simulink model "DriveFinal"  (R2023a)
settings: Solver=FixedStepDiscrete  StartTime=0.0  StopTime=10.0  FixedStep=0.01  RelTol=1e-3
undefined symbols (not defined in the file): InputPWM, WheelSpeed
libraries: mobileRoboticsTrainingLib x5
settings Model: Creator=Jack Youens  LastModifiedBy=jakew

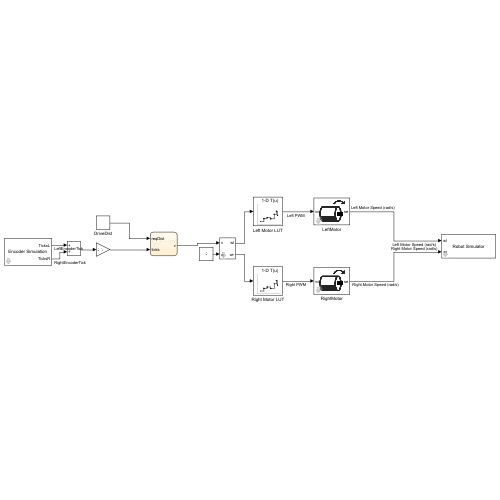
[thumbnail: Simulink's stored preview of the top-level diagram]
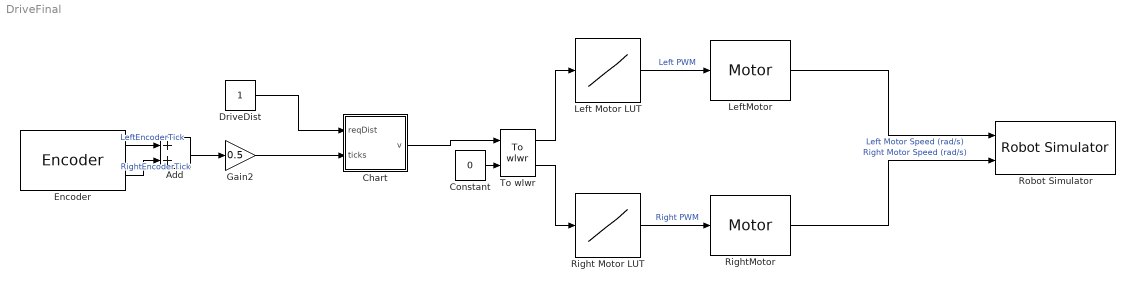
== system DriveFinal ==
  Add : Sum
  Chart : Stateflow chart  TreatAsAtomicUnit=on
  Constant : Constant  Value=0
  DriveDist : Constant
  Encoder : mobileRoboticsTrainingLib/Encoder  axleLength=axleLength  wheelR=wheelR  ticksPerRot=ticksPerRot
      settings: SourceProductName=Mobile Robotics Training Library
  Gain2 : Gain  Gain=0.5
  Left Motor LUT : Lookup_n-D  NumberOfTableDimensions=1  BreakpointsForDimension1=WheelSpeed  Table=InputPWM  InterpMethod=Nearest  ExtrapMethod=Clip  InternalRulePriority=Speed  RndMeth=Simplest
  LeftMotor : mobileRoboticsTrainingLib/Motor  motorPlant=wheelMotorModel  sensorType=Speed
      settings: SourceProductName=Mobile Robotics Training Library
  Right Motor LUT : Lookup_n-D  NumberOfTableDimensions=1  BreakpointsForDimension1=WheelSpeed  Table=InputPWM  InterpMethod=Nearest  ExtrapMethod=Clip  InternalRulePriority=Speed  RndMeth=Simplest
  RightMotor : mobileRoboticsTrainingLib/Motor  motorPlant=wheelMotorModel  sensorType=Speed
      settings: SourceProductName=Mobile Robotics Training Library
  Robot Simulator : mobileRoboticsTrainingLib/Robot Simulator  Priority=99  mapVar=mapForSim  startX=0.5  startY=0.1  startTheta=90  axleLength=axleLength  wheelR=wheelR
  To wlwr : mobileRoboticsTrainingLib/To wlwr  axleLength=0.1  wheelR=0.05
      link override change parameters: Gain=[1 -axleLength/2; 1 axleLength/2]
  wires:
  DriveDist/1 -> Chart/1(reqDist)
  Add/1 -> Gain2/1
  LeftMotor/1 -> Robot Simulator/1  "Left Motor Speed (rad/s)"
  To wlwr/2 -> Right Motor LUT/1
  To wlwr/1 -> Left Motor LUT/1
  Right Motor LUT/1 -> RightMotor/1  "Right PWM"
  RightMotor/1 -> Robot Simulator/2  "Right Motor Speed (rad/s)"
  Left Motor LUT/1 -> LeftMotor/1  "Left PWM"
  Constant/1 -> To wlwr/2
  Chart/1(v) -> To wlwr/1
  Encoder/2 -> Add/2  "RightEncoderTick"
  Encoder/1 -> Add/1  "LeftEncoderTick"
  Gain2/1 -> Chart/2(ticks)

== stateflow chart DriveFinal/Chart ==
  state Default
    entry:
    ticks;
    dist1Tick=(pi*0.031)/10
    reqTicks=reqDist/dist1Tick;
  state Stop
    entry:
    v=0;
  state Move
    entry:
    v=0.5;
  (default) -> Default
  Default -> Stop [order 2] : [ticks==reqTicks | ticks>reqTicks]
  Move -> Default
  Default -> Move [order 1] : [ticks<reqTicks]
  data: reqDist input; ticks input; v output; dist1Tick local; reqTicks local
